simulink model "phan1_bai3b_2016"  (R2019a)
settings: Solver=VariableStepAuto  StartTime=0.0  StopTime=60  RelTol=1e-3
libraries: simulink x1
settings Model: Creator=inhuo  LastModifiedBy=inhuo
settings OptimizationCC: LifeSpan=inf
settings DebuggingCC: ArithmeticOperatorsInVariantConditions=warning
settings CodeAppCC: StateflowObjectComments=on

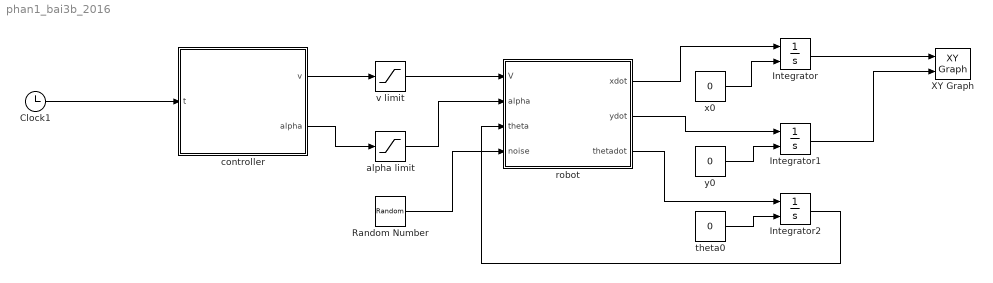
== system phan1_bai3b_2016 ==
  Clock1 : Clock
  Integrator : Integrator  InitialConditionSource=external
  Integrator1 : Integrator  InitialConditionSource=external
  Integrator2 : Integrator  InitialConditionSource=external
  Random Number : RandomNumber  Variance=pi/36  SampleTime=0.01
  XY Graph : simulink/Sinks/XY Graph  xmin=-1  xmax=25  ymin=-10  ymax=1  st=-1
  alpha limit : Saturate  UpperLimit=pi/4  LowerLimit=-pi/4
  controller : MATLAB Function  TreatAsAtomicUnit=on
  "robot " : MATLAB Function  TreatAsAtomicUnit=on
  theta0 : Constant  Value=0
  "v limit " : Saturate  UpperLimit=1.83  LowerLimit=-1.83
  x0 : Constant  Value=0
  y0 : Constant  Value=0
  wires:
  "v limit "/1 -> "robot "/1(V)
  controller/2(alpha) -> alpha limit/1
  "robot "/1(xdot) -> Integrator/1
  alpha limit/1 -> "robot "/2(alpha)
  x0/1 -> Integrator/2
  Integrator/1 -> XY Graph/1
  y0/1 -> Integrator1/2
  Clock1/1 -> controller/1(t)
  "robot "/3(thetadot) -> Integrator2/1
  Integrator1/1 -> XY Graph/2
  "robot "/2(ydot) -> Integrator1/1
  theta0/1 -> Integrator2/2
  controller/1(v) -> "v limit "/1
  Integrator2/1 -> "robot "/3(theta)
  Random Number/1 -> "robot "/4(noise)

== matlab function phan1_bai3b_2016/controller ==
  data: v output; t input; alpha output
function [v, alpha] = fcn(t)
    % Setup Config
    G = 9;
    d = sqrt(2.5 + 0.1*G); % Axial Space
    
    if t < 20
        v = 1;
        alpha = 0;
    elseif (t >= 20) && ( t<= 40)
        v = pi/5;    
        alpha = -atan2(d, 4);
    elseif (t >= 41) && (t <= 61)
        v = 1;
        alpha = 0;
    else
        v = 0;
        alpha = 0;
    end
end

== matlab function phan1_bai3b_2016/robot  ==
  data: V input; xdot output; alpha input; theta input; ydot output; thetadot output; noise input
function [xdot , ydot , thetadot]= fcn(V,alpha,theta,noise)
    d = sqrt(2.5 + 0.1*9); 

    % Kinematic Equations
    xdot = V * cos(theta);
    ydot = V * sin(theta);
    thetadot = V * tan(alpha + noise)/d;
end

% case 1 
% xdot = V*cos(alpha)*cos(theta);
% ydot = V*cos(alpha)*sin(theta);
% thetadot =V*sin(alpha)/d;

% case 2
% xdot = V*cos(theta);
% ydot = V*sin(theta);
% thetadot =V*tan(alpha)/d;
